simulink model "Ekstrapolacja"  (R2022b)
settings: Solver=VariableStepAuto  StartTime=0.0  StopTime=20  RelTol=1e-3
values from neighbouring files (symbols this model uses):
  Ts = 0.15    [PID_TEMPERATURA.m]    (also in PID_proj.m = 0.01)
undefined symbols (not defined in the file or in its folder): DiscIntNeverNeededParam, SensTs
libraries: slpidlib x2
settings Model: Creator=hpiet  LastModifiedBy=hpiet

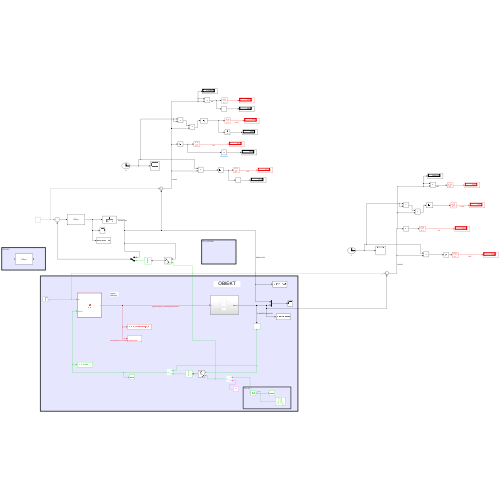
[thumbnail: Simulink's stored preview of the top-level diagram]
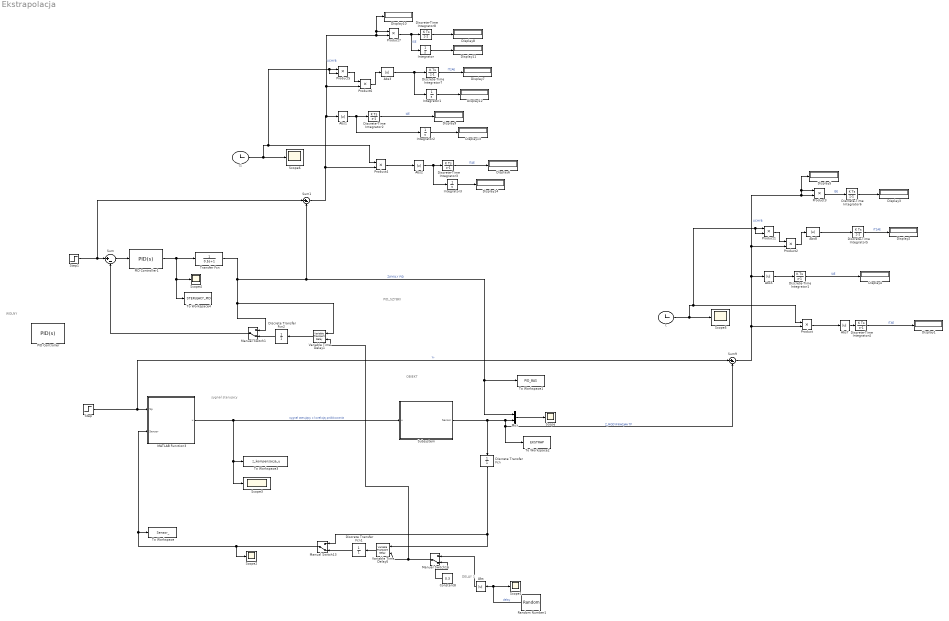
== system Ekstrapolacja ==
  note: WOLNY
  note: PID_SZYBKI
  note: sygnał sterujacy
  note: OBIEKT
  note: DELAY 1
  Abs{,1..3,5,7..8} (7 alike) : Abs  SaturateOnIntegerOverflow=off
  Constant8 : Constant  Value=0.3
  Discrete Transfer Fcn : DiscreteTransferFcn  Denominator=[1]  SampleTime=SensTs
  Discrete Transfer Fcn1 : DiscreteTransferFcn  Denominator=[1]  SampleTime=SensTs
  Discrete Transfer Fcn2 : DiscreteTransferFcn  Denominator=[1]  SampleTime=SensTs
  Discrete-Time Integrator{1..8} (8 alike) : DiscreteIntegrator  SampleTime=Ts  ICPrevOutput=DiscIntNeverNeededParam  ICPrevScaledInput=DiscIntNeverNeededParam
  Display{1..14} (14 alike) : Display
  Integrator{,1..3} (4 alike) : Integrator
  MATLAB Function3 : MATLAB Function  TreatAsAtomicUnit=on  SystemSampleTime=0.01
  Manual Switch1 : ManualSwitch  CurrentSetting=0
  Manual Switch13 : ManualSwitch  CurrentSetting=0
  Manual Switch16 : ManualSwitch  CurrentSetting=0
  Mux : Mux  Inputs=2
  PID Controller : slpidlib/PID Controller  Controller=PID  Form=Parallel  TimeDomain=Continuous-time  UseExternalTs=off  SampleTime=-1  IntegratorMethod=Forward Euler  FilterMethod=Forward Euler  ControllerParametersSource=internal  P=0.170660134954593  I=0.00995973814137223  UseKiTs=off  D=0.113784041827361  N=0.811881285656632  UseFilter=on  TunerSelectOption=Transfer Function Based (PID Tuner App)  InitialConditionSource=internal  InitialConditionForIntegrator=0  InitialConditionForFilter=0  DifferentiatorICPrevScaledInput=0  ExternalReset=none  TrackingMode=off  Kt=1  LimitOutput=off  SatLimitsSource=internal  UpperSaturationLimit=inf  LowerSaturationLimit=-inf  LinearizeAsGain=on  AntiWindupMode=none  Kb=1  LimitIntegrator=off  UpperIntegratorSaturationLimit=inf  LowerIntegratorSaturationLimit=-inf  POutMin=[]  POutMax=[]  IOutMin=[]  IOutMax=[]  DOutMin=[]  DOutMax=[]  NOutMin=[]  NOutMax=[]  SumOutMin=[]  SumOutMax=[]  SaturationOutMin=[]  SaturationOutMax=[]  PParamMin=[]  PParamMax=[]  IParamMin=[]  IParamMax=[]  DParamMin=[]  DParamMax=[]  NParamMin=[]  NParamMax=[]  KbParamMin=[]  KbParamMax=[]  KtParamMin=[]  KtParamMax=[]  KbOutMin=[]  KbOutMax=[]  KtOutMin=[]  KtOutMax=[]  IntegratorOutMin=[]  IntegratorOutMax=[]  FilterOutMin=[]  FilterOutMax=[]  SumI1OutMin=[]  SumI1OutMax=[]  SumI2OutMin=[]  SumI2OutMax=[]  SumI3OutMin=[]  SumI3OutMax=[]  SumI4OutMin=[]  SumI4OutMax=[]  SumDOutMin=[]  SumDOutMax=[]  DifferentiatorOutMin=[]  DifferentiatorOutMax=[]  FilterDiffOutCoefMin=[]  FilterDiffOutCoefMax=[]  ReciprocalOutMin=[]  ReciprocalOutMax=[]  SumDenOutMin=[]  SumDenOutMax=[]  SumNumOutMin=[]  SumNumOutMax=[]  DivideOutMin=[]  DivideOutMax=[]  UdiffTsProdOutMin=[]  UdiffTsProdOutMax=[]  NTsProdOutMin=[]  NTsProdOutMax=[]  UintegralTsProdOutMin=[]  UintegralTsProdOutMax=[]  UngainTsProdOutMin=[]  UngainTsProdOutMax=[]  ClampingZeroOutDataTypeStr=Inherit: Inherit via back propagation  ClampingZeroOutMin=[]  ClampingZeroOutMax=[]  FilterDenConstantOutDataTypeStr=Inherit: Inherit via back propagation  FilterDenConstantOutMin=[]  FilterDenConstantOutMax=[]  PCopyOutDataTypeStr=Inherit: Inherit via back propagation  PCopyOutMin=[]  PCopyOutMax=[]  NCopyOutDataTypeStr=Inherit: Inherit via back propagation  NCopyOutMin=[]  NCopyOutMax=[]  IntegratorContinuousStateAttributes=''  IntegratorStateMustResolveToSignalObject=off  IntegratorRTWStateStorageClass=Auto  FilterContinuousStateAttributes=''  FilterStateMustResolveToSignalObject=off  FilterRTWStateStorageClass=Auto  ParallelPVariant=InternalParameters  IdealPVariant=Disabled  IVariant=InternalParameters  DVariant=InternalParameters  IntegratorVariant=Continuous  SatVariant=Disabled  AWVariant=Passthrough  PCopyVariant=Disabled  TRVariant=Disabled  FdbkBlocksVariant=Forward  IdealPFdbkVariant=Disabled  SatFdbkVariant=Disabled  DerivativeFilterVariant=ContFilter  NVariant=InternalParameters  NCopyVariant=Disabled  FilterICVariant=InternalICsFilter  IntegratorICVariant=InternalICs  ExternalResetVariant=Disabled  TRSumVariant=Passthrough  SumFdbkVariant=Disabled  SumVariant=Sum_PID  TsampFilterVariant=InternalTs  TsampNgainVariant=Passthrough  TsampIntegralVariant=Passthrough  ExternalSaturationOutDataTypeStr=Inherit: Same as second input
  PID Controller1 : slpidlib/PID Controller  Controller=PID  Form=Parallel  TimeDomain=Continuous-time  UseExternalTs=off  SampleTime=-1  IntegratorMethod=Forward Euler  FilterMethod=Forward Euler  ControllerParametersSource=internal  P=0.352652053728451;  I=0.477399324378819;  UseKiTs=off  D=0  N=0.588685123145228;  UseFilter=on  TunerSelectOption=Transfer Function Based (PID Tuner App)  InitialConditionSource=internal  InitialConditionForIntegrator=0  InitialConditionForFilter=0  DifferentiatorICPrevScaledInput=0  ExternalReset=none  TrackingMode=off  Kt=1  LimitOutput=off  SatLimitsSource=internal  UpperSaturationLimit=inf  LowerSaturationLimit=-inf  LinearizeAsGain=on  AntiWindupMode=none  Kb=1  LimitIntegrator=off  UpperIntegratorSaturationLimit=inf  LowerIntegratorSaturationLimit=-inf  POutMin=[]  POutMax=[]  IOutMin=[]  IOutMax=[]  DOutMin=[]  DOutMax=[]  NOutMin=[]  NOutMax=[]  SumOutMin=[]  SumOutMax=[]  SaturationOutMin=[]  SaturationOutMax=[]  PParamMin=[]  PParamMax=[]  IParamMin=[]  IParamMax=[]  DParamMin=[]  DParamMax=[]  NParamMin=[]  NParamMax=[]  KbParamMin=[]  KbParamMax=[]  KtParamMin=[]  KtParamMax=[]  KbOutMin=[]  KbOutMax=[]  KtOutMin=[]  KtOutMax=[]  IntegratorOutMin=[]  IntegratorOutMax=[]  FilterOutMin=[]  FilterOutMax=[]  SumI1OutMin=[]  SumI1OutMax=[]  SumI2OutMin=[]  SumI2OutMax=[]  SumI3OutMin=[]  SumI3OutMax=[]  SumI4OutMin=[]  SumI4OutMax=[]  SumDOutMin=[]  SumDOutMax=[]  DifferentiatorOutMin=[]  DifferentiatorOutMax=[]  FilterDiffOutCoefMin=[]  FilterDiffOutCoefMax=[]  ReciprocalOutMin=[]  ReciprocalOutMax=[]  SumDenOutMin=[]  SumDenOutMax=[]  SumNumOutMin=[]  SumNumOutMax=[]  DivideOutMin=[]  DivideOutMax=[]  UdiffTsProdOutMin=[]  UdiffTsProdOutMax=[]  NTsProdOutMin=[]  NTsProdOutMax=[]  UintegralTsProdOutMin=[]  UintegralTsProdOutMax=[]  UngainTsProdOutMin=[]  UngainTsProdOutMax=[]  ClampingZeroOutDataTypeStr=Inherit: Inherit via back propagation  ClampingZeroOutMin=[]  ClampingZeroOutMax=[]  FilterDenConstantOutDataTypeStr=Inherit: Inherit via back propagation  FilterDenConstantOutMin=[]  FilterDenConstantOutMax=[]  PCopyOutDataTypeStr=Inherit: Inherit via back propagation  PCopyOutMin=[]  PCopyOutMax=[]  NCopyOutDataTypeStr=Inherit: Inherit via back propagation  NCopyOutMin=[]  NCopyOutMax=[]  IntegratorContinuousStateAttributes=''  IntegratorStateMustResolveToSignalObject=off  IntegratorRTWStateStorageClass=Auto  FilterContinuousStateAttributes=''  FilterStateMustResolveToSignalObject=off  FilterRTWStateStorageClass=Auto  ParallelPVariant=InternalParameters  IdealPVariant=Disabled  IVariant=InternalParameters  DVariant=InternalParameters  IntegratorVariant=Continuous  SatVariant=Disabled  AWVariant=Passthrough  PCopyVariant=Disabled  TRVariant=Disabled  FdbkBlocksVariant=Forward  IdealPFdbkVariant=Disabled  SatFdbkVariant=Disabled  DerivativeFilterVariant=ContFilter  NVariant=InternalParameters  NCopyVariant=Disabled  FilterICVariant=InternalICsFilter  IntegratorICVariant=InternalICs  ExternalResetVariant=Disabled  TRSumVariant=Passthrough  SumFdbkVariant=Disabled  SumVariant=Sum_PID  TsampFilterVariant=InternalTs  TsampNgainVariant=Passthrough  TsampIntegralVariant=Passthrough  ExternalSaturationOutDataTypeStr=Inherit: Same as second input
  Product{,1..7} (8 alike) : Product
  Random Number1 : RandomNumber  Mean=0.5  Variance=0.0001  SampleTime=0.5
  Scope{,1..6} (7 alike) : Scope
  Step : Step  Time=0  After=25
  Step1 : Step  Time=0  After=25
  Subsystem : Subsystem
  Sum : Sum  Inputs=|+-
  Sum1 : Sum  Inputs=|+-
  Sum9 : Sum  Inputs=|+-
  To Workspace : ToWorkspace  VariableName=Sensor_  SaveFormat=Timeseries  SampleTime=-1
  To Workspace1 : ToWorkspace  VariableName=PID_BAS  SaveFormat=Timeseries  SampleTime=-1
  To Workspace2 : ToWorkspace  VariableName=EKSTRAP  SaveFormat=Timeseries  SampleTime=-1
  To Workspace3 : ToWorkspace  VariableName=z_kompensacja_u  SaveFormat=Timeseries  SampleTime=-1
  To Workspace4 : ToWorkspace  VariableName=STERUJACY_PID  SaveFormat=Timeseries  SampleTime=-1
  Transfer Fcn : TransferFcn  Denominator=[0.5 1]
  Variable Time Delay1 : VariableTransportDelay  MaximumDelay=1000
  Variable Time Delay5 : VariableTransportDelay  MaximumDelay=1000
  t : Clock
  t1 : Clock
  wires:
  Random Number1/1 -> Scope1/1, Abs/1  "delay"
  Subsystem/1(Sensor) -> Sum9/2, To Workspace2/1, Mux/2, Discrete Transfer Fcn/1  "Z_MODYFIKACJAA TP"
  Variable Time Delay5/1 -> Discrete Transfer Fcn1/1
  Constant8/1 -> Manual Switch16/2
  Discrete Transfer Fcn/1 -> Manual Switch13/1, Variable Time Delay5/1
  Discrete Transfer Fcn1/1 -> Manual Switch13/2
  MATLAB Function3/1(u) -> Subsystem/1(u), Scope3/1, To Workspace3/1  "sygnał sterujący z korekcją próbkowania"
  Manual Switch13/1 -> To Workspace/1, MATLAB Function3/2(Sensor), Scope2/1
  Step1/1 -> Sum1/1, Sum/1
  Sum/1 -> PID Controller1/1
  PID Controller1/1 -> Scope4/1, To Workspace4/1, Transfer Fcn/1
  Transfer Fcn/1 -> Sum1/2, To Workspace1/1, Mux/1, Variable Time Delay1/1, Manual Switch1/1  "ZWYKŁY PID"
  Manual Switch16/1 -> Variable Time Delay1/2, Variable Time Delay5/2
  Variable Time Delay1/1 -> Discrete Transfer Fcn2/1
  Discrete Transfer Fcn2/1 -> Manual Switch1/2
  Manual Switch1/1 -> Sum/2
  Mux/1 -> Scope/1
  Abs/1 -> Manual Switch16/1
  Product2/1 -> Abs8/1
  Discrete-Time Integrator4/1 -> Display1/1  "ITAE"
  Discrete-Time Integrator5/1 -> Display2/1  "IT2AE"
  Product3/1 -> Discrete-Time Integrator6/1  "ISE"
  Discrete-Time Integrator6/1 -> Display3/1
  Abs7/1 -> Discrete-Time Integrator4/1
  Sum9/1 -> Product/2, Product2/2, Display5/1, Product3/1, Product3/2, Abs5/1  "UCHYB"
  Product1/1 -> Product2/1
  Abs8/1 -> Discrete-Time Integrator5/1
  Abs5/1 -> Discrete-Time Integrator1/1
  Step/1 -> Sum9/1, MATLAB Function3/1(Sp)  "Yr"
  Discrete-Time Integrator1/1 -> Display4/1  "IAE"
  Product/1 -> Abs7/1
  t/1 -> Product1/2, Product1/1, Product/1, Scope5/1
  t1/1 -> Product5/2, Product5/1, Product4/1, Scope6/1
  Product4/1 -> Abs2/1
  Product5/1 -> Product6/1
  Sum1/1 -> Product4/2, Product6/2, Display10/1, Product7/1, Product7/2, Abs1/1  "UCHYB"
  Discrete-Time Integrator8/1 -> Display8/1
  Discrete-Time Integrator7/1 -> Display7/1  "IT2AE"
  Discrete-Time Integrator2/1 -> Display9/1  "IAE"
  Discrete-Time Integrator3/1 -> Display6/1  "ITAE"
  Product6/1 -> Abs3/1
  Abs1/1 -> Integrator2/1, Discrete-Time Integrator2/1
  Product7/1 -> Integrator/1, Discrete-Time Integrator8/1  "ISE"
  Abs3/1 -> Integrator1/1, Discrete-Time Integrator7/1
  Abs2/1 -> Integrator3/1, Discrete-Time Integrator3/1
  Integrator/1 -> Display11/1
  Integrator1/1 -> Display12/1
  Integrator2/1 -> Display13/1
  Integrator3/1 -> Display14/1

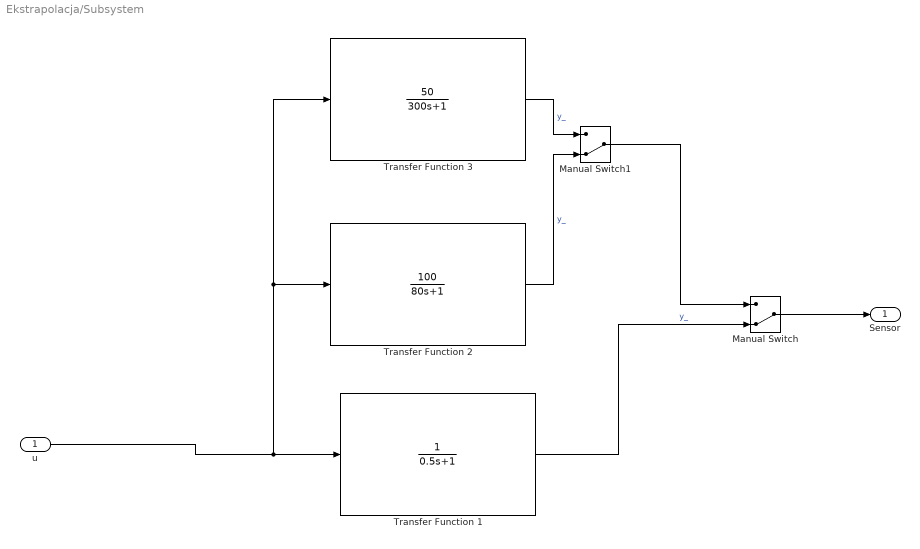
== system Ekstrapolacja/Subsystem ==
  u : Inport
  Manual Switch : ManualSwitch  CurrentSetting=0
  Manual Switch1 : ManualSwitch  CurrentSetting=0
  Transfer Function 1 : TransferFcn  Denominator=[0.5 1]
  Transfer Function 2 : TransferFcn  Numerator=[100]  Denominator=[80 1]
  Transfer Function 3 : TransferFcn  Numerator=[50]  Denominator=[300 1]
  Sensor : Outport
  wires:
  u/1 -> Transfer Function 3/1, Transfer Function 2/1, Transfer Function 1/1
  Transfer Function 1/1 -> Manual Switch/2  "y_"
  Manual Switch/1 -> Sensor/1
  Transfer Function 3/1 -> Manual Switch1/1  "y_"
  Manual Switch1/1 -> Manual Switch/1
  Transfer Function 2/1 -> Manual Switch1/2  "y_"

== matlab function Ekstrapolacja/MATLAB Function3 ==
  settings: updateMethod=DISCRETE
  data: Sp input; u output; Sensor input
function u = fcn(Sp,Sensor) %wyjscie = funkcja(wejscia)
persistent init e2 e1 u2 u1 ku1 ku2 ke0 ke1 ke2 pomiar czas Ts vec_czas przewidywaniex N;

if isempty(init) %wykonuje się tylko raz


%NASTAWY : OBIEKT 100/80s+1

% Kp = 1.50833;
% Ki =0.0031789;
% Kd = 2.9488110947;
% FCoef = 0.121320071;

%NASTAWY: OBIEKT 1/100s+1

% Kp = 4.00784874415517;
% Ki =0.0905840820709279;
% Kd = 10.3091445576305;
% FCoef = 0.0532104379131174;
% 


%OBIEKT WOLNY

% Kp=0.170660134954593;
% Ki=0.00995973814137223;
% Kd=0.113784041827361;
% FCoef=0.811881285656632;

%OBIEKT SZYBKI

Kp = 0.352652053728451;
Ki =0.477399324378819;
Kd = 0;
FCoef = 0.588685123145228;

Ts=0.01; %czas próbki


e2=0;
e1=0;
u2=0;
u1=0;

%DO EKSTRAPOLACJI

pomiar = Sensor;
czas = 0;
vec_czas = 0;
przewidywaniex=0;

%TEMPORARY TEST
N=0; %500 pomiarów zaczyna sie ekstrapolacja

%TEST
a0 = (1 + FCoef * Ts);
a1 = -(2 + FCoef * Ts);
a2 = 1;

b0=Kp*(1+FCoef * Ts) + Ki*Ts*(1+ FCoef*Ts) + Kd*FCoef;
b1= -(Kp*(2+FCoef*Ts) + Ki*Ts + 2*Kd*FCoef);
b2=Kp + Kd * FCoef;

%uproszczenie równania
ku1=a1/a0;
ku2=a2/a0;
ke0=b0/a0;
ke1=b1/a0;
ke2=b2/a0;

init=1;


%TMP TEST
end

%EKSTRAPOLACJA PROBEK

czas=czas+0.5;
vec_czas = [vec_czas,czas];
pomiar = [pomiar, Sensor];

disp('dlugosc wektora czasu')
disp(size(vec_czas,2))
disp(vec_czas(end))
disp('aktualny czas')
disp(czas)

disp('ilosc pomiarow')
disp(size(pomiar,2))



if(N<50 || mod(N,50))  % Pierwsze 500 próbek a następnie wykonywane co 5 próbkę

    e0 = Sp-Sensor;
    u0 = -(ku1*u1) - (ku2 * u2) + (ke0*e0) + (ke1*e1) + (ke2*e2);

    e2=e1;
    e1=e0;
    u2=u1;
    u1=u0;

    u=u0;

elseif(N>=50) % ROZPOCZĘCIE EKSTRAPOLACJI

    ekstrapolacjax = linspace( vec_czas(end-2), vec_czas(end)+0.5 ,10000);

    przewidywaniex = interp1(vec_czas,pomiar,ekstrapolacjax,'linear','extrap');
    disp(przewidywaniex);


    e0 = Sp-przewidywaniex(end);
    u0 = -(ku1*u1) - (ku2 * u2) + (ke0*e0) + (ke1*e1) + (ke2*e2);

    e2=e1;
    e1=e0;
    u2=u1;
    u1=u0;

    u=u0;

else 
    u=0; % gdy to wyrzucę to mamy błąd

end

N=N+1;
end
